simulink model "ProcessAccelerometer"  (R2020a)
settings: Solver=FixedStepAuto  StartTime=0.0  StopTime=10.0  FixedStep=1e-3  RelTol=1e-3  EnableMultiTasking=on
libraries: frdmk64flib x4, simulink x3
settings Model: ExtModeTrigDuration=5  Creator=WinnieTrandinh  LastModifiedBy=WinnieTrandinh
settings OptimizationCC: EnhancedBackFolding=on  PassReuseOutputArgsAs=Individual arguments  ZeroExternalMemoryAtStartup=off  ZeroInternalMemoryAtStartup=off  MaxStackSize=64  OptimizeBlockOrder=speed  DifferentSizesBufferReuse=on  OptimizationCustomize=off  EfficientTunableParamExpr=on
settings DebuggingCC: ParameterTunabilityLossMsg=error
settings HardwareCC: ProdBitPerPointer=32  ProdBitPerSizeT=32  ProdBitPerPtrDiffT=32  ProdLargestAtomicInteger=Long  ProdLargestAtomicFloat=Double  ProdWordSize=32  ProdHWDeviceType=ARM Compatible->ARM Cortex
settings SFSimCC: MATLABDynamicMemAlloc=off
settings RTWCC: SystemTargetFile=ert.tlc  HardwareBoard=NXP FRDM-K64F  TemplateMakefile=ert_default_tmf  Toolchain=GNU Tools for ARM Embedded Processors
settings CodeAppCC: ForceParamTrailComments=on  IgnoreCustomStorageClasses=off  OperatorAnnotations=on  SimulinkDataObjDesc=on  SFDataObjDesc=on  InsertBlockDesc=on

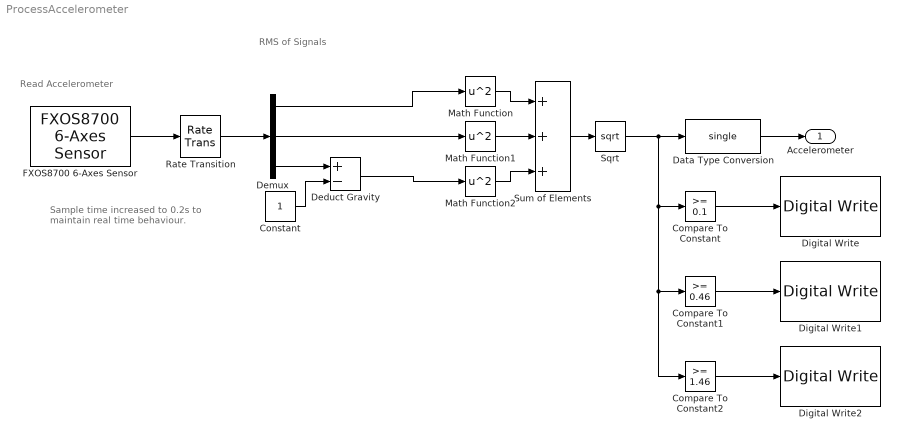
== system ProcessAccelerometer ==
  note: RMS of Signals
  note: Sample time increased to 0.2s to
      | maintain real time behaviour.
  note: Read Accelerometer
  Compare To Constant : simulink/Logic and Bit Operations/Compare To Constant  relop=>=  const=0.1  OutDataTypeStr=boolean
  Compare To Constant1 : simulink/Logic and Bit Operations/Compare To Constant  relop=>=  const=0.46  OutDataTypeStr=boolean
  Compare To Constant2 : simulink/Logic and Bit Operations/Compare To Constant  relop=>=  const=1.46  OutDataTypeStr=boolean
  Constant : Constant
  Data Type Conversion : DataTypeConversion  OutDataTypeStr=single
  Deduct Gravity : Sum  Inputs=+-
  Demux : Demux  Outputs=3
  Digital Write : frdmk64flib/Digital Write  Whichpin=RED_LED
  Digital Write1 : frdmk64flib/Digital Write  Whichpin=GREEN_LED
  Digital Write2 : frdmk64flib/Digital Write  Whichpin=BLUE_LED
  FXOS8700 6-Axes Sensor : frdmk64flib/FXOS8700 6-Axes Sensor  Activesensor=Accelerometer only  ODR=400Hz  HybridODR=400Hz  Accelfullrange=-2g to +2g  SampleTime=0.2
  Math Function : Math  Operator=square  SaturateOnIntegerOverflow=on
  Math Function1 : Math  Operator=square  SaturateOnIntegerOverflow=on
  Math Function2 : Math  Operator=square  SaturateOnIntegerOverflow=on
  Rate Transition : RateTransition
  Sqrt : Sqrt  SaturateOnIntegerOverflow=on
  Sum of Elements : Sum  Inputs=+++
  Accelerometer : Outport  OutDataTypeStr=single
  wires:
  Deduct Gravity/1 -> Math Function2/1
  Demux/1 -> Math Function/1
  Constant/1 -> Deduct Gravity/2
  Math Function/1 -> Sum of Elements/1
  Math Function1/1 -> Sum of Elements/2
  Math Function2/1 -> Sum of Elements/3
  Compare To Constant/1 -> Digital Write/1
  Compare To Constant1/1 -> Digital Write1/1
  Compare To Constant2/1 -> Digital Write2/1
  Demux/3 -> Deduct Gravity/1
  Demux/2 -> Math Function1/1
  Sqrt/1 -> Compare To Constant2/1, Compare To Constant1/1, Compare To Constant/1, Data Type Conversion/1
  Sum of Elements/1 -> Sqrt/1
  FXOS8700 6-Axes Sensor/1 -> Rate Transition/1
  Rate Transition/1 -> Demux/1
  Data Type Conversion/1 -> Accelerometer/1
